simulink model "ROPOD_Control_SIM"  (R2017b)
settings: Solver=VariableStepAuto  StartTime=0.0  StopTime=inf  RelTol=1e-3
values from neighbouring files (symbols this model uses):
  AgentNumber = 1    [init_model.m]
  FFtheta_intia = 0    [init_model.m]
  FFxy_mass = 0*80    (= 0)    [init_model.m]
  flock_FFtheta_friction = 50    [init_model.m]
  flock_FFxy_friction = 100    [init_model.m]
  I_fhz_ddelta_cntr = 0    [init_model.m]
  I_fhz_dtheta_cntr = 0.3    [init_model.m]
  I_fhz_dtheta_flock_cntr = 0.1    [init_model.m]
  I_fhz_dvarphi_cntr = 0    [init_model.m]
  I_fhz_dxdy_cntr = 0.25    [init_model.m]
  I_fhz_dxdy_flock_cntr = 0.1    [init_model.m]
  K_gain_ddelta_cntr = 0.1    [init_model.m]
  K_gain_dtheta_cntr = 150    [init_model.m]
  K_gain_dtheta_flock_cntr = 100    [init_model.m]
  K_gain_dvarphi_cntr = 0.05    [init_model.m]
  K_gain_dxdy_cntr = 200    [init_model.m]
  K_gain_dxdy_flock_cntr = 200    [init_model.m]
  LL_wp_fhz_ddelta_cntr = 2    [init_model.m]
  LL_wp_fhz_dtheta_cntr = 20    [init_model.m]
  LL_wp_fhz_dtheta_flock_cntr = 20    [init_model.m]
  LL_wp_fhz_dvarphi_cntr = 10    [init_model.m]
  LL_wp_fhz_dxdy_cntr = 20    [init_model.m]
  LL_wp_fhz_dxdy_flock_cntr = 20    [init_model.m]
  LL_wz_fhz_ddelta_cntr = 2    [init_model.m]
  LL_wz_fhz_dtheta_cntr = 20    [init_model.m]
  LL_wz_fhz_dtheta_flock_cntr = 20    [init_model.m]
  LL_wz_fhz_dvarphi_cntr = 2    [init_model.m]
  LL_wz_fhz_dxdy_cntr = 20    [init_model.m]
  LL_wz_fhz_dxdy_flock_cntr = 20    [init_model.m]
  LPF_fhz_ddelta_cntr = 50    [init_model.m]
  LPF_fhz_ddelta_meas = 50    [init_model.m]
  LPF_fhz_dtheta_cntr = 100    [init_model.m]
  LPF_fhz_dtheta_flock_cntr = 40    [init_model.m]
  LPF_fhz_dvarphi_cntr = 50    [init_model.m]
  LPF_fhz_dvarphi_meas = 50    [init_model.m]
  LPF_fhz_dxdy_cntr = 100    [init_model.m]
  LPF_fhz_dxdy_flock_cntr = 40    [init_model.m]
  max_flock_acc_theta = 0.5    [init_model.m]
  max_flock_acc_xy = 0.5    [init_model.m]
  max_flock_vel_theta = 1.0    (= 1)    [init_model.m]
  max_flock_vel_xy = 1.0    (= 1)    [init_model.m]
  max_hw_tau = 7.0    (= 7)    [init_model.m]
  max_ropod_acc_theta = 1.6    [init_model.m]
  max_ropod_acc_xy = 2.0    (= 2)    [init_model.m]
  max_ropod_sw_force = 500    [init_model.m]
  max_ropod_sw_tau = 250    [init_model.m]
  max_ropod_vel_theta = 1.6    [init_model.m]
  max_ropod_vel_xy = 2.0    (= 2)    [init_model.m]
  max_sw_current = 10    [init_model.m]
  Nagents = 2    [init_model.m]
  Nwheels = 4    [Jqwl_numeric_function.m]    (also in S_matrix.m; extract_kinmodel_parameters.m; init_model.m; tau_optimal_dist_vec_fun.m)
  pivot_offs_sws = [0.0243    0.4689    0.3384    5.9050]    [init_model.m]
  ropod_kinmodel_pv = struct2array(ropod_kinmodel_param)    [set_ropod_KinModparams.m]
  ropod_position_inflock = [-1 0 3.1416]    [init_model.m]
  SW_COM1_ENABLE1 = hex2dec('0001')    [init_model.m]
  SW_COM1_ENABLE2 = hex2dec('0002')    [init_model.m]
  SW_COM1_MODE_TORQUE = bitshift(hex2dec('0000'),2)    [init_model.m]
  SW_COM1_MODE_VELOCITY = bitshift(hex2dec('0002'),2)    [init_model.m]
  SW_COM1_USE_TS = hex2dec('8000')    [init_model.m]
  sw_tau_2_current = 1/motor_physical_parameters.torqueconstant.value    [init_model.m]
  Tinit = 2    [init_model.m]
  Ts = 0.001    [init_model.m]
  Ts_MPC = 0.01    [init_model.m]
  Tsflck = 0.01    [init_model.m]
undefined symbols (not defined in the file or in its folder): acc_limit, accmax, b_cx, b_cy, b_rx, bus_size, comp_enable, Desired, DiscIntNeverNeededParam, Fcgain, gdis, k_cx, k_cy, live_tuning, m_robot, Nominal, Nominal_x, Nominal_y, offsets, portwidth, sizes, types, vel_limit, vmax1, vmax2
libraries: simulink x90, cstblocks x66, dspsigops x12, dspnetwork x4
(part 5 of 8)

== system ROPOD_Control_SIM/FlockController/Flock Velocity controller/G_I_LL_LPF Controller_flock_Y/Shapeit Lead-Lag (Tustin) ==
  In : Inport
  fz : Inport  Port=2
  fp : Inport  Port=3
  Add : Sum  Inputs=+-
  Constant1 : Constant
  Constant2 : Constant  Value=0
  Constant4 : Constant
  Divide : Product  Inputs=*/
  Divide1 : Product  Inputs=/*
  Gain1 : Gain  Gain=2*pi
  Gain2 : Gain  Gain=2*pi
  PID Controller3 : simulink/Continuous/PID Controller  Controller=PID  TimeDomain=Discrete-time  SampleTime=Tsflck  IntegratorMethod=Trapezoidal  FilterMethod=Trapezoidal  Form=Parallel  UseFilter=on  ControllerParametersSource=external  P=0.4  I=0.4*2*pi*3  D=0  N=100  InitialConditionSource=internal  InitialConditionForIntegrator=0  InitialConditionForFilter=0  ExternalReset=none  LimitOutput=off  UpperSaturationLimit=max_hw_tau  LowerSaturationLimit=-max_hw_tau  LinearizeAsGain=on  AntiWindupMode=clamping  Kb=1  TrackingMode=off  Kt=1  PParamMin=[]  PParamMax=[]  IParamMin=[]  IParamMax=[]  DParamMin=[]  DParamMax=[]  NParamMin=[]  NParamMax=[]  KbParamMin=[]  KbParamMax=[]  KtParamMin=[]  KtParamMax=[]  POutMin=[]  POutMax=[]  IOutMin=[]  IOutMax=[]  DOutMin=[]  DOutMax=[]  NOutMin=[]  NOutMax=[]  KbOutMin=[]  KbOutMax=[]  KtOutMin=[]  KtOutMax=[]  IntegratorOutMin=[]  IntegratorOutMax=[]  FilterOutMin=[]  FilterOutMax=[]  SumOutMin=[]  SumOutMax=[]  SumI1OutMin=[]  SumI1OutMax=[]  SumI2OutMin=[]  SumI2OutMax=[]  SumI3OutMin=[]  SumI3OutMax=[]  SumDOutMin=[]  SumDOutMax=[]  SaturationOutMin=[]  SaturationOutMax=[]  IntegratorContinuousStateAttributes=''  IntegratorStateMustResolveToSignalObject=off  IntegratorRTWStateStorageClass=Auto  FilterContinuousStateAttributes=''  FilterStateMustResolveToSignalObject=off  FilterRTWStateStorageClass=Auto  DifferentiatorICPrevScaledInput=0  DifferentiatorOutMin=[]  DifferentiatorOutMax=[]  InitialConditionSetting=State (most efficient)  FilterDiffOutCoefMin=[]  FilterDiffOutCoefMax=[]  SumDenOutMin=[]  SumDenOutMax=[]  SumNumOutMin=[]  SumNumOutMax=[]  ReciprocalOutMin=[]  ReciprocalOutMax=[]  DivideOutMin=[]  DivideOutMax=[]  TunerSelectOption=Transfer Function Based (PID Tuner App)
  Out : Outport
  wires:
  Constant4/1 -> PID Controller3/2
  In/1 -> PID Controller3/1
  PID Controller3/1 -> Out/1
  fz/1 -> Gain2/1
  fp/1 -> Gain1/1
  Gain1/1 -> PID Controller3/5, Divide/2
  Constant2/1 -> PID Controller3/3
  Gain2/1 -> Divide1/1, Divide/1
  Divide/1 -> Add/2
  Constant1/1 -> Add/1
  Add/1 -> Divide1/2
  Divide1/1 -> PID Controller3/4

== system ROPOD_Control_SIM/RopodTorqueDistribution/ROPOD 4SW/ROPOD_4Wheel_sens_own_vel_filter/Glitch removal + LP filter ==
  encoder : Inport
  LPF_fhz : Inport  Port=2
  Constant3 : Constant  Value=Ts
  Discrete Derivative : simulink/Discrete/Discrete Derivative  gainval=1  ICPrevScaledInput=0.0  OutMin=[]  OutMax=[]  OutDataType=fixdt(1, 16)  OutScaling=2^-10  DoSatur=off
  Discrete Varying Lowpass12 : cstblocks/Linear Parameter Varying/Discrete Varying Lowpass  N=2  w0=0  Ts=Ts
      settings: SourceProductName=Control System Toolbox  SourceProductBaseCode=CT
  Remove_glitches1 : MATLAB Function  TreatAsAtomicUnit=on
  Unit Delay : UnitDelay  SampleTime=-1
  Unwrap11 : dspsigops/Unwrap  tol=0.1  running=on
  sign convention4 : Gain  Gain=2*pi
  out : Outport
  wires:
  Unit Delay/1 -> Remove_glitches1/1(vel)
  sign convention4/1 -> Discrete Varying Lowpass12/2
  Unwrap11/1 -> Remove_glitches1/3(encoder)
  LPF_fhz/1 -> sign convention4/1
  Remove_glitches1/1(encoder_out) -> Discrete Derivative/1
  Constant3/1 -> Remove_glitches1/2(Ts)
  Discrete Varying Lowpass12/1 -> out/1
  encoder/1 -> Unwrap11/1
  Discrete Derivative/1 -> Unit Delay/1, Discrete Varying Lowpass12/1

== system ROPOD_Control_SIM/RopodTorqueDistribution/ROPOD 4SW/ROPOD_4Wheel_sens_own_vel_filter/Glitch removal + LP filter1 ==
  encoder : Inport
  LPF_fhz : Inport  Port=2
  Constant3 : Constant  Value=Ts
  Discrete Derivative : simulink/Discrete/Discrete Derivative  gainval=1  ICPrevScaledInput=0.0  OutMin=[]  OutMax=[]  OutDataType=fixdt(1, 16)  OutScaling=2^-10  DoSatur=off
  Discrete Varying Lowpass12 : cstblocks/Linear Parameter Varying/Discrete Varying Lowpass  N=2  w0=0  Ts=Ts
      settings: SourceProductName=Control System Toolbox  SourceProductBaseCode=CT
  Remove_glitches1 : MATLAB Function  TreatAsAtomicUnit=on
  Unit Delay : UnitDelay  SampleTime=-1
  Unwrap11 : dspsigops/Unwrap  tol=0.1  running=on
  sign convention4 : Gain  Gain=2*pi
  out : Outport
  wires:
  Discrete Derivative/1 -> Discrete Varying Lowpass12/1, Unit Delay/1
  encoder/1 -> Unwrap11/1
  Discrete Varying Lowpass12/1 -> out/1
  Constant3/1 -> Remove_glitches1/2(Ts)
  Remove_glitches1/1(encoder_out) -> Discrete Derivative/1
  LPF_fhz/1 -> sign convention4/1
  Unwrap11/1 -> Remove_glitches1/3(encoder)
  sign convention4/1 -> Discrete Varying Lowpass12/2
  Unit Delay/1 -> Remove_glitches1/1(vel)

== system ROPOD_Control_SIM/RopodTorqueDistribution/ROPOD 4SW/ROPOD_4Wheel_sens_own_vel_filter/Glitch removal + LP filter10 ==
  encoder : Inport
  LPF_fhz : Inport  Port=2
  Constant3 : Constant  Value=Ts
  Discrete Derivative : simulink/Discrete/Discrete Derivative  gainval=1  ICPrevScaledInput=0.0  OutMin=[]  OutMax=[]  OutDataType=fixdt(1, 16)  OutScaling=2^-10  DoSatur=off
  Discrete Varying Lowpass12 : cstblocks/Linear Parameter Varying/Discrete Varying Lowpass  N=2  w0=0  Ts=Ts
      settings: SourceProductName=Control System Toolbox  SourceProductBaseCode=CT
  Remove_glitches1 : MATLAB Function  TreatAsAtomicUnit=on
  Unit Delay : UnitDelay  SampleTime=-1
  Unwrap11 : dspsigops/Unwrap  tol=0.1  running=on
  sign convention4 : Gain  Gain=2*pi
  enc_out : Outport
  out : Outport  Port=2
  wires:
  Unit Delay/1 -> Remove_glitches1/1(vel)
  sign convention4/1 -> Discrete Varying Lowpass12/2
  Unwrap11/1 -> Remove_glitches1/3(encoder)
  LPF_fhz/1 -> sign convention4/1
  Remove_glitches1/1(encoder_out) -> enc_out/1, Discrete Derivative/1
  Constant3/1 -> Remove_glitches1/2(Ts)
  Discrete Varying Lowpass12/1 -> out/1
  encoder/1 -> Unwrap11/1
  Discrete Derivative/1 -> Unit Delay/1, Discrete Varying Lowpass12/1

== system ROPOD_Control_SIM/RopodTorqueDistribution/ROPOD 4SW/ROPOD_4Wheel_sens_own_vel_filter/Glitch removal + LP filter11 ==
  encoder : Inport
  LPF_fhz : Inport  Port=2
  Constant3 : Constant  Value=Ts
  Discrete Derivative : simulink/Discrete/Discrete Derivative  gainval=1  ICPrevScaledInput=0.0  OutMin=[]  OutMax=[]  OutDataType=fixdt(1, 16)  OutScaling=2^-10  DoSatur=off
  Discrete Varying Lowpass12 : cstblocks/Linear Parameter Varying/Discrete Varying Lowpass  N=2  w0=0  Ts=Ts
      settings: SourceProductName=Control System Toolbox  SourceProductBaseCode=CT
  Remove_glitches1 : MATLAB Function  TreatAsAtomicUnit=on
  Unit Delay : UnitDelay  SampleTime=-1
  Unwrap11 : dspsigops/Unwrap  tol=0.1  running=on
  sign convention4 : Gain  Gain=2*pi
  encoder_out : Outport
  vel_out : Outport  Port=2
  wires:
  Unit Delay/1 -> Remove_glitches1/1(vel)
  sign convention4/1 -> Discrete Varying Lowpass12/2
  Unwrap11/1 -> Remove_glitches1/3(encoder)
  LPF_fhz/1 -> sign convention4/1
  Remove_glitches1/1(encoder_out) -> encoder_out/1, Discrete Derivative/1
  Constant3/1 -> Remove_glitches1/2(Ts)
  Discrete Varying Lowpass12/1 -> vel_out/1
  encoder/1 -> Unwrap11/1
  Discrete Derivative/1 -> Unit Delay/1, Discrete Varying Lowpass12/1

== system ROPOD_Control_SIM/RopodTorqueDistribution/ROPOD 4SW/ROPOD_4Wheel_sens_own_vel_filter/Glitch removal + LP filter2 ==
  encoder : Inport
  LPF_fhz : Inport  Port=2
  Constant3 : Constant  Value=Ts
  Discrete Derivative : simulink/Discrete/Discrete Derivative  gainval=1  ICPrevScaledInput=0.0  OutMin=[]  OutMax=[]  OutDataType=fixdt(1, 16)  OutScaling=2^-10  DoSatur=off
  Discrete Varying Lowpass12 : cstblocks/Linear Parameter Varying/Discrete Varying Lowpass  N=2  w0=0  Ts=Ts
      settings: SourceProductName=Control System Toolbox  SourceProductBaseCode=CT
  Remove_glitches1 : MATLAB Function  TreatAsAtomicUnit=on
  Unit Delay : UnitDelay  SampleTime=-1
  Unwrap11 : dspsigops/Unwrap  tol=0.1  running=on
  sign convention4 : Gain  Gain=2*pi
  encoder_out : Outport
  vel_out : Outport  Port=2
  wires:
  Unit Delay/1 -> Remove_glitches1/1(vel)
  sign convention4/1 -> Discrete Varying Lowpass12/2
  Unwrap11/1 -> Remove_glitches1/3(encoder)
  LPF_fhz/1 -> sign convention4/1
  Remove_glitches1/1(encoder_out) -> encoder_out/1, Discrete Derivative/1
  Constant3/1 -> Remove_glitches1/2(Ts)
  Discrete Varying Lowpass12/1 -> vel_out/1
  encoder/1 -> Unwrap11/1
  Discrete Derivative/1 -> Unit Delay/1, Discrete Varying Lowpass12/1

== system ROPOD_Control_SIM/RopodTorqueDistribution/ROPOD 4SW/ROPOD_4Wheel_sens_own_vel_filter/Glitch removal + LP filter3 ==
  encoder : Inport
  LPF_fhz : Inport  Port=2
  Constant3 : Constant  Value=Ts
  Discrete Derivative : simulink/Discrete/Discrete Derivative  gainval=1  ICPrevScaledInput=0.0  OutMin=[]  OutMax=[]  OutDataType=fixdt(1, 16)  OutScaling=2^-10  DoSatur=off
  Discrete Varying Lowpass12 : cstblocks/Linear Parameter Varying/Discrete Varying Lowpass  N=2  w0=0  Ts=Ts
      settings: SourceProductName=Control System Toolbox  SourceProductBaseCode=CT
  Remove_glitches1 : MATLAB Function  TreatAsAtomicUnit=on
  Unit Delay : UnitDelay  SampleTime=-1
  Unwrap11 : dspsigops/Unwrap  tol=0.1  running=on
  sign convention4 : Gain  Gain=2*pi
  out : Outport
  wires:
  Unit Delay/1 -> Remove_glitches1/1(vel)
  sign convention4/1 -> Discrete Varying Lowpass12/2
  Unwrap11/1 -> Remove_glitches1/3(encoder)
  LPF_fhz/1 -> sign convention4/1
  Remove_glitches1/1(encoder_out) -> Discrete Derivative/1
  Constant3/1 -> Remove_glitches1/2(Ts)
  Discrete Varying Lowpass12/1 -> out/1
  encoder/1 -> Unwrap11/1
  Discrete Derivative/1 -> Unit Delay/1, Discrete Varying Lowpass12/1

== system ROPOD_Control_SIM/RopodTorqueDistribution/ROPOD 4SW/ROPOD_4Wheel_sens_own_vel_filter/Glitch removal + LP filter4 ==
  encoder : Inport
  LPF_fhz : Inport  Port=2
  Constant3 : Constant  Value=Ts
  Discrete Derivative : simulink/Discrete/Discrete Derivative  gainval=1  ICPrevScaledInput=0.0  OutMin=[]  OutMax=[]  OutDataType=fixdt(1, 16)  OutScaling=2^-10  DoSatur=off
  Discrete Varying Lowpass12 : cstblocks/Linear Parameter Varying/Discrete Varying Lowpass  N=2  w0=0  Ts=Ts
      settings: SourceProductName=Control System Toolbox  SourceProductBaseCode=CT
  Remove_glitches1 : MATLAB Function  TreatAsAtomicUnit=on
  Unit Delay : UnitDelay  SampleTime=-1
  Unwrap11 : dspsigops/Unwrap  tol=0.1  running=on
  sign convention4 : Gain  Gain=2*pi
  out : Outport
  wires:
  Discrete Derivative/1 -> Discrete Varying Lowpass12/1, Unit Delay/1
  encoder/1 -> Unwrap11/1
  Discrete Varying Lowpass12/1 -> out/1
  Constant3/1 -> Remove_glitches1/2(Ts)
  Remove_glitches1/1(encoder_out) -> Discrete Derivative/1
  LPF_fhz/1 -> sign convention4/1
  Unwrap11/1 -> Remove_glitches1/3(encoder)
  sign convention4/1 -> Discrete Varying Lowpass12/2
  Unit Delay/1 -> Remove_glitches1/1(vel)

== system ROPOD_Control_SIM/RopodTorqueDistribution/ROPOD 4SW/ROPOD_4Wheel_sens_own_vel_filter/Glitch removal + LP filter5 ==
  encoder : Inport
  LPF_fhz : Inport  Port=2
  Constant3 : Constant  Value=Ts
  Discrete Derivative : simulink/Discrete/Discrete Derivative  gainval=1  ICPrevScaledInput=0.0  OutMin=[]  OutMax=[]  OutDataType=fixdt(1, 16)  OutScaling=2^-10  DoSatur=off
  Discrete Varying Lowpass12 : cstblocks/Linear Parameter Varying/Discrete Varying Lowpass  N=2  w0=0  Ts=Ts
      settings: SourceProductName=Control System Toolbox  SourceProductBaseCode=CT
  Remove_glitches1 : MATLAB Function  TreatAsAtomicUnit=on
  Unit Delay : UnitDelay  SampleTime=-1
  Unwrap11 : dspsigops/Unwrap  tol=0.1  running=on
  sign convention4 : Gain  Gain=2*pi
  encoder_out : Outport
  vel_out : Outport  Port=2
  wires:
  Unit Delay/1 -> Remove_glitches1/1(vel)
  sign convention4/1 -> Discrete Varying Lowpass12/2
  Unwrap11/1 -> Remove_glitches1/3(encoder)
  LPF_fhz/1 -> sign convention4/1
  Remove_glitches1/1(encoder_out) -> encoder_out/1, Discrete Derivative/1
  Constant3/1 -> Remove_glitches1/2(Ts)
  Discrete Varying Lowpass12/1 -> vel_out/1
  encoder/1 -> Unwrap11/1
  Discrete Derivative/1 -> Unit Delay/1, Discrete Varying Lowpass12/1

== system ROPOD_Control_SIM/RopodTorqueDistribution/ROPOD 4SW/ROPOD_4Wheel_sens_own_vel_filter/Glitch removal + LP filter6 ==
  encoder : Inport
  LPF_fhz : Inport  Port=2
  Constant3 : Constant  Value=Ts
  Discrete Derivative : simulink/Discrete/Discrete Derivative  gainval=1  ICPrevScaledInput=0.0  OutMin=[]  OutMax=[]  OutDataType=fixdt(1, 16)  OutScaling=2^-10  DoSatur=off
  Discrete Varying Lowpass12 : cstblocks/Linear Parameter Varying/Discrete Varying Lowpass  N=2  w0=0  Ts=Ts
      settings: SourceProductName=Control System Toolbox  SourceProductBaseCode=CT
  Remove_glitches1 : MATLAB Function  TreatAsAtomicUnit=on
  Unit Delay : UnitDelay  SampleTime=-1
  Unwrap11 : dspsigops/Unwrap  tol=0.1  running=on
  sign convention4 : Gain  Gain=2*pi
  out : Outport
  wires:
  Unit Delay/1 -> Remove_glitches1/1(vel)
  sign convention4/1 -> Discrete Varying Lowpass12/2
  Unwrap11/1 -> Remove_glitches1/3(encoder)
  LPF_fhz/1 -> sign convention4/1
  Remove_glitches1/1(encoder_out) -> Discrete Derivative/1
  Constant3/1 -> Remove_glitches1/2(Ts)
  Discrete Varying Lowpass12/1 -> out/1
  encoder/1 -> Unwrap11/1
  Discrete Derivative/1 -> Unit Delay/1, Discrete Varying Lowpass12/1

== system ROPOD_Control_SIM/RopodTorqueDistribution/ROPOD 4SW/ROPOD_4Wheel_sens_own_vel_filter/Glitch removal + LP filter7 ==
  encoder : Inport
  LPF_fhz : Inport  Port=2
  Constant3 : Constant  Value=Ts
  Discrete Derivative : simulink/Discrete/Discrete Derivative  gainval=1  ICPrevScaledInput=0.0  OutMin=[]  OutMax=[]  OutDataType=fixdt(1, 16)  OutScaling=2^-10  DoSatur=off
  Discrete Varying Lowpass12 : cstblocks/Linear Parameter Varying/Discrete Varying Lowpass  N=2  w0=0  Ts=Ts
      settings: SourceProductName=Control System Toolbox  SourceProductBaseCode=CT
  Remove_glitches1 : MATLAB Function  TreatAsAtomicUnit=on
  Unit Delay : UnitDelay  SampleTime=-1
  Unwrap11 : dspsigops/Unwrap  tol=0.1  running=on
  sign convention4 : Gain  Gain=2*pi
  out : Outport
  wires:
  Discrete Derivative/1 -> Discrete Varying Lowpass12/1, Unit Delay/1
  encoder/1 -> Unwrap11/1
  Discrete Varying Lowpass12/1 -> out/1
  Constant3/1 -> Remove_glitches1/2(Ts)
  Remove_glitches1/1(encoder_out) -> Discrete Derivative/1
  LPF_fhz/1 -> sign convention4/1
  Unwrap11/1 -> Remove_glitches1/3(encoder)
  sign convention4/1 -> Discrete Varying Lowpass12/2
  Unit Delay/1 -> Remove_glitches1/1(vel)

== system ROPOD_Control_SIM/RopodTorqueDistribution/ROPOD 4SW/ROPOD_4Wheel_sens_own_vel_filter/Glitch removal + LP filter8 ==
  encoder : Inport
  LPF_fhz : Inport  Port=2
  Constant3 : Constant  Value=Ts
  Discrete Derivative : simulink/Discrete/Discrete Derivative  gainval=1  ICPrevScaledInput=0.0  OutMin=[]  OutMax=[]  OutDataType=fixdt(1, 16)  OutScaling=2^-10  DoSatur=off
  Discrete Varying Lowpass12 : cstblocks/Linear Parameter Varying/Discrete Varying Lowpass  N=2  w0=0  Ts=Ts
      settings: SourceProductName=Control System Toolbox  SourceProductBaseCode=CT
  Remove_glitches1 : MATLAB Function  TreatAsAtomicUnit=on
  Unit Delay : UnitDelay  SampleTime=-1
  Unwrap11 : dspsigops/Unwrap  tol=0.1  running=on
  sign convention4 : Gain  Gain=2*pi
  encoder_out : Outport
  vel_out : Outport  Port=2
  wires:
  Unit Delay/1 -> Remove_glitches1/1(vel)
  sign convention4/1 -> Discrete Varying Lowpass12/2
  Unwrap11/1 -> Remove_glitches1/3(encoder)
  LPF_fhz/1 -> sign convention4/1
  Remove_glitches1/1(encoder_out) -> encoder_out/1, Discrete Derivative/1
  Constant3/1 -> Remove_glitches1/2(Ts)
  Discrete Varying Lowpass12/1 -> vel_out/1
  encoder/1 -> Unwrap11/1
  Discrete Derivative/1 -> Unit Delay/1, Discrete Varying Lowpass12/1

== system ROPOD_Control_SIM/RopodTorqueDistribution/ROPOD 4SW/ROPOD_4Wheel_sens_own_vel_filter/Glitch removal + LP filter9 ==
  encoder : Inport
  LPF_fhz : Inport  Port=2
  Constant3 : Constant  Value=Ts
  Discrete Derivative : simulink/Discrete/Discrete Derivative  gainval=1  ICPrevScaledInput=0.0  OutMin=[]  OutMax=[]  OutDataType=fixdt(1, 16)  OutScaling=2^-10  DoSatur=off
  Discrete Varying Lowpass12 : cstblocks/Linear Parameter Varying/Discrete Varying Lowpass  N=2  w0=0  Ts=Ts
      settings: SourceProductName=Control System Toolbox  SourceProductBaseCode=CT
  Remove_glitches1 : MATLAB Function  TreatAsAtomicUnit=on
  Unit Delay : UnitDelay  SampleTime=-1
  Unwrap11 : dspsigops/Unwrap  tol=0.1  running=on
  sign convention4 : Gain  Gain=2*pi
  enc_out : Outport
  out : Outport  Port=2
  wires:
  Unit Delay/1 -> Remove_glitches1/1(vel)
  sign convention4/1 -> Discrete Varying Lowpass12/2
  Unwrap11/1 -> Remove_glitches1/3(encoder)
  LPF_fhz/1 -> sign convention4/1
  Remove_glitches1/1(encoder_out) -> enc_out/1, Discrete Derivative/1
  Constant3/1 -> Remove_glitches1/2(Ts)
  Discrete Varying Lowpass12/1 -> out/1
  encoder/1 -> Unwrap11/1
  Discrete Derivative/1 -> Unit Delay/1, Discrete Varying Lowpass12/1

== system ROPOD_Control_SIM/RopodTorqueDistribution/pivot damping cntr/Pivot controller/G_I_LL_LPF Controller1 ==
  param : Inport
  In : Inport  Port=2
  reset_integrator : Inport  Port=3
  Bus Selector : BusSelector  OutputSignals=P_gain,I_freq_hz,LL_zero_fhz,LL_pole_fhz,LPF_fhz
  Discrete Varying Lowpass3 : cstblocks/Linear Parameter Varying/Discrete Varying Lowpass  N=1  w0=0  Ts=Ts
      settings: SourceProductName=Control System Toolbox  SourceProductBaseCode=CT
  Gain2 : Gain  Gain=2*pi
  Product5 : Product
  Shapeit Integrator (Tustin) : Subsystem
  Shapeit Lead-Lag (Tustin) : Subsystem
  Out : Outport
  wires:
  Gain2/1 -> Discrete Varying Lowpass3/2
  Product5/1 -> Shapeit Integrator (Tustin)/1(In)
  Discrete Varying Lowpass3/1 -> Out/1
  Shapeit Integrator (Tustin)/1(Out) -> Shapeit Lead-Lag (Tustin)/1(In)
  Bus Selector/1 -> Product5/2  "<P_gain>"
  Bus Selector/2 -> Shapeit Integrator (Tustin)/2(I_fhz)  "<I_freq_hz>"
  param/1 -> Bus Selector/1
  Bus Selector/5 -> Gain2/1  "<LPF_fhz>"
  Bus Selector/4 -> Shapeit Lead-Lag (Tustin)/3(fp)  "<LL_pole_fhz>"
  reset_integrator/1 -> Shapeit Integrator (Tustin)/3(reset)
  Bus Selector/3 -> Shapeit Lead-Lag (Tustin)/2(fz)  "<LL_zero_fhz>"
  Shapeit Lead-Lag (Tustin)/1(Out) -> Discrete Varying Lowpass3/1
  In/1 -> Product5/1

== system ROPOD_Control_SIM/RopodTorqueDistribution/pivot damping cntr/Pivot controller/G_I_LL_LPF Controller2 ==
  param : Inport
  In : Inport  Port=2
  reset_integrator : Inport  Port=3
  Bus Selector : BusSelector  OutputSignals=P_gain,I_freq_hz,LL_zero_fhz,LL_pole_fhz,LPF_fhz
  Discrete Varying Lowpass3 : cstblocks/Linear Parameter Varying/Discrete Varying Lowpass  N=1  w0=0  Ts=Ts
      settings: SourceProductName=Control System Toolbox  SourceProductBaseCode=CT
  Gain2 : Gain  Gain=2*pi
  Product5 : Product
  Shapeit Integrator (Tustin) : Subsystem
  Shapeit Lead-Lag (Tustin) : Subsystem
  Out : Outport
  wires:
  Gain2/1 -> Discrete Varying Lowpass3/2
  Product5/1 -> Shapeit Integrator (Tustin)/1(In)
  Discrete Varying Lowpass3/1 -> Out/1
  Shapeit Integrator (Tustin)/1(Out) -> Shapeit Lead-Lag (Tustin)/1(In)
  Bus Selector/1 -> Product5/2  "<P_gain>"
  Bus Selector/2 -> Shapeit Integrator (Tustin)/2(I_fhz)  "<I_freq_hz>"
  param/1 -> Bus Selector/1
  Bus Selector/5 -> Gain2/1  "<LPF_fhz>"
  Bus Selector/4 -> Shapeit Lead-Lag (Tustin)/3(fp)  "<LL_pole_fhz>"
  reset_integrator/1 -> Shapeit Integrator (Tustin)/3(reset)
  Bus Selector/3 -> Shapeit Lead-Lag (Tustin)/2(fz)  "<LL_zero_fhz>"
  Shapeit Lead-Lag (Tustin)/1(Out) -> Discrete Varying Lowpass3/1
  In/1 -> Product5/1

== system ROPOD_Control_SIM/RopodTorqueDistribution/pivot damping cntr/Pivot controller/G_I_LL_LPF Controller3 ==
  param : Inport
  In : Inport  Port=2
  reset_integrator : Inport  Port=3
  Bus Selector : BusSelector  OutputSignals=P_gain,I_freq_hz,LL_zero_fhz,LL_pole_fhz,LPF_fhz
  Discrete Varying Lowpass3 : cstblocks/Linear Parameter Varying/Discrete Varying Lowpass  N=1  w0=0  Ts=Ts
      settings: SourceProductName=Control System Toolbox  SourceProductBaseCode=CT
  Gain2 : Gain  Gain=2*pi
  Product5 : Product
  Shapeit Integrator (Tustin) : Subsystem
  Shapeit Lead-Lag (Tustin) : Subsystem
  Out : Outport
  wires:
  In/1 -> Product5/1
  Shapeit Lead-Lag (Tustin)/1(Out) -> Discrete Varying Lowpass3/1
  Bus Selector/3 -> Shapeit Lead-Lag (Tustin)/2(fz)  "<LL_zero_fhz>"
  reset_integrator/1 -> Shapeit Integrator (Tustin)/3(reset)
  Bus Selector/4 -> Shapeit Lead-Lag (Tustin)/3(fp)  "<LL_pole_fhz>"
  Bus Selector/5 -> Gain2/1  "<LPF_fhz>"
  param/1 -> Bus Selector/1
  Bus Selector/2 -> Shapeit Integrator (Tustin)/2(I_fhz)  "<I_freq_hz>"
  Bus Selector/1 -> Product5/2  "<P_gain>"
  Shapeit Integrator (Tustin)/1(Out) -> Shapeit Lead-Lag (Tustin)/1(In)
  Discrete Varying Lowpass3/1 -> Out/1
  Product5/1 -> Shapeit Integrator (Tustin)/1(In)
  Gain2/1 -> Discrete Varying Lowpass3/2

== system ROPOD_Control_SIM/RopodTorqueDistribution/pivot damping cntr/Pivot controller/G_I_LL_LPF Controller4 ==
  param : Inport
  In : Inport  Port=2
  reset_integrator : Inport  Port=3
  Bus Selector : BusSelector  OutputSignals=P_gain,I_freq_hz,LL_zero_fhz,LL_pole_fhz,LPF_fhz
  Discrete Varying Lowpass3 : cstblocks/Linear Parameter Varying/Discrete Varying Lowpass  N=1  w0=0  Ts=Ts
      settings: SourceProductName=Control System Toolbox  SourceProductBaseCode=CT
  Gain2 : Gain  Gain=2*pi
  Product5 : Product
  Shapeit Integrator (Tustin) : Subsystem
  Shapeit Lead-Lag (Tustin) : Subsystem
  Out : Outport
  wires:
  Gain2/1 -> Discrete Varying Lowpass3/2
  Product5/1 -> Shapeit Integrator (Tustin)/1(In)
  Discrete Varying Lowpass3/1 -> Out/1
  Shapeit Integrator (Tustin)/1(Out) -> Shapeit Lead-Lag (Tustin)/1(In)
  Bus Selector/1 -> Product5/2  "<P_gain>"
  Bus Selector/2 -> Shapeit Integrator (Tustin)/2(I_fhz)  "<I_freq_hz>"
  param/1 -> Bus Selector/1
  Bus Selector/5 -> Gain2/1  "<LPF_fhz>"
  Bus Selector/4 -> Shapeit Lead-Lag (Tustin)/3(fp)  "<LL_pole_fhz>"
  reset_integrator/1 -> Shapeit Integrator (Tustin)/3(reset)
  Bus Selector/3 -> Shapeit Lead-Lag (Tustin)/2(fz)  "<LL_zero_fhz>"
  Shapeit Lead-Lag (Tustin)/1(Out) -> Discrete Varying Lowpass3/1
  In/1 -> Product5/1

== system ROPOD_Control_SIM/RopodTorqueDistribution/wheel vel cntr/Wheels Velocity controller/G_I_LL_LPF Controller1 ==
  param : Inport
  In : Inport  Port=2
  reset_integrator : Inport  Port=3
  Bus Selector : BusSelector  OutputSignals=P_gain,I_freq_hz,LL_zero_fhz,LL_pole_fhz,LPF_fhz
  Discrete Varying Lowpass3 : cstblocks/Linear Parameter Varying/Discrete Varying Lowpass  N=1  w0=0  Ts=Ts
      settings: SourceProductName=Control System Toolbox  SourceProductBaseCode=CT
  Gain2 : Gain  Gain=2*pi
  Product5 : Product
  Shapeit Integrator (Tustin) : Subsystem
  Shapeit Lead-Lag (Tustin) : Subsystem
  Out : Outport
  wires:
  Gain2/1 -> Discrete Varying Lowpass3/2
  Product5/1 -> Shapeit Integrator (Tustin)/1(In)
  Discrete Varying Lowpass3/1 -> Out/1
  Shapeit Integrator (Tustin)/1(Out) -> Shapeit Lead-Lag (Tustin)/1(In)
  Bus Selector/1 -> Product5/2  "<P_gain>"
  Bus Selector/2 -> Shapeit Integrator (Tustin)/2(I_fhz)  "<I_freq_hz>"
  param/1 -> Bus Selector/1
  Bus Selector/5 -> Gain2/1  "<LPF_fhz>"
  Bus Selector/4 -> Shapeit Lead-Lag (Tustin)/3(fp)  "<LL_pole_fhz>"
  reset_integrator/1 -> Shapeit Integrator (Tustin)/3(reset)
  Bus Selector/3 -> Shapeit Lead-Lag (Tustin)/2(fz)  "<LL_zero_fhz>"
  Shapeit Lead-Lag (Tustin)/1(Out) -> Discrete Varying Lowpass3/1
  In/1 -> Product5/1

== system ROPOD_Control_SIM/RopodTorqueDistribution/wheel vel cntr/Wheels Velocity controller/G_I_LL_LPF Controller2 ==
  param : Inport
  In : Inport  Port=2
  reset_integrator : Inport  Port=3
  Bus Selector : BusSelector  OutputSignals=P_gain,I_freq_hz,LL_zero_fhz,LL_pole_fhz,LPF_fhz
  Discrete Varying Lowpass3 : cstblocks/Linear Parameter Varying/Discrete Varying Lowpass  N=1  w0=0  Ts=Ts
      settings: SourceProductName=Control System Toolbox  SourceProductBaseCode=CT
  Gain2 : Gain  Gain=2*pi
  Product5 : Product
  Shapeit Integrator (Tustin) : Subsystem
  Shapeit Lead-Lag (Tustin) : Subsystem
  Out : Outport
  wires:
  Gain2/1 -> Discrete Varying Lowpass3/2
  Product5/1 -> Shapeit Integrator (Tustin)/1(In)
  Discrete Varying Lowpass3/1 -> Out/1
  Shapeit Integrator (Tustin)/1(Out) -> Shapeit Lead-Lag (Tustin)/1(In)
  Bus Selector/1 -> Product5/2  "<P_gain>"
  Bus Selector/2 -> Shapeit Integrator (Tustin)/2(I_fhz)  "<I_freq_hz>"
  param/1 -> Bus Selector/1
  Bus Selector/5 -> Gain2/1  "<LPF_fhz>"
  Bus Selector/4 -> Shapeit Lead-Lag (Tustin)/3(fp)  "<LL_pole_fhz>"
  reset_integrator/1 -> Shapeit Integrator (Tustin)/3(reset)
  Bus Selector/3 -> Shapeit Lead-Lag (Tustin)/2(fz)  "<LL_zero_fhz>"
  Shapeit Lead-Lag (Tustin)/1(Out) -> Discrete Varying Lowpass3/1
  In/1 -> Product5/1

== system ROPOD_Control_SIM/RopodTorqueDistribution/wheel vel cntr/Wheels Velocity controller/G_I_LL_LPF Controller3 ==
  param : Inport
  In : Inport  Port=2
  reset_integrator : Inport  Port=3
  Bus Selector : BusSelector  OutputSignals=P_gain,I_freq_hz,LL_zero_fhz,LL_pole_fhz,LPF_fhz
  Discrete Varying Lowpass3 : cstblocks/Linear Parameter Varying/Discrete Varying Lowpass  N=1  w0=0  Ts=Ts
      settings: SourceProductName=Control System Toolbox  SourceProductBaseCode=CT
  Gain2 : Gain  Gain=2*pi
  Product5 : Product
  Shapeit Integrator (Tustin) : Subsystem
  Shapeit Lead-Lag (Tustin) : Subsystem
  Out : Outport
  wires:
  In/1 -> Product5/1
  Shapeit Lead-Lag (Tustin)/1(Out) -> Discrete Varying Lowpass3/1
  Bus Selector/3 -> Shapeit Lead-Lag (Tustin)/2(fz)  "<LL_zero_fhz>"
  reset_integrator/1 -> Shapeit Integrator (Tustin)/3(reset)
  Bus Selector/4 -> Shapeit Lead-Lag (Tustin)/3(fp)  "<LL_pole_fhz>"
  Bus Selector/5 -> Gain2/1  "<LPF_fhz>"
  param/1 -> Bus Selector/1
  Bus Selector/2 -> Shapeit Integrator (Tustin)/2(I_fhz)  "<I_freq_hz>"
  Bus Selector/1 -> Product5/2  "<P_gain>"
  Shapeit Integrator (Tustin)/1(Out) -> Shapeit Lead-Lag (Tustin)/1(In)
  Discrete Varying Lowpass3/1 -> Out/1
  Product5/1 -> Shapeit Integrator (Tustin)/1(In)
  Gain2/1 -> Discrete Varying Lowpass3/2

== system ROPOD_Control_SIM/RopodTorqueDistribution/wheel vel cntr/Wheels Velocity controller/G_I_LL_LPF Controller4 ==
  param : Inport
  In : Inport  Port=2
  reset_integrator : Inport  Port=3
  Bus Selector : BusSelector  OutputSignals=P_gain,I_freq_hz,LL_zero_fhz,LL_pole_fhz,LPF_fhz
  Discrete Varying Lowpass3 : cstblocks/Linear Parameter Varying/Discrete Varying Lowpass  N=1  w0=0  Ts=Ts
      settings: SourceProductName=Control System Toolbox  SourceProductBaseCode=CT
  Gain2 : Gain  Gain=2*pi
  Product5 : Product
  Shapeit Integrator (Tustin) : Subsystem
  Shapeit Lead-Lag (Tustin) : Subsystem
  Out : Outport
  wires:
  Gain2/1 -> Discrete Varying Lowpass3/2
  Product5/1 -> Shapeit Integrator (Tustin)/1(In)
  Discrete Varying Lowpass3/1 -> Out/1
  Shapeit Integrator (Tustin)/1(Out) -> Shapeit Lead-Lag (Tustin)/1(In)
  Bus Selector/1 -> Product5/2  "<P_gain>"
  Bus Selector/2 -> Shapeit Integrator (Tustin)/2(I_fhz)  "<I_freq_hz>"
  param/1 -> Bus Selector/1
  Bus Selector/5 -> Gain2/1  "<LPF_fhz>"
  Bus Selector/4 -> Shapeit Lead-Lag (Tustin)/3(fp)  "<LL_pole_fhz>"
  reset_integrator/1 -> Shapeit Integrator (Tustin)/3(reset)
  Bus Selector/3 -> Shapeit Lead-Lag (Tustin)/2(fz)  "<LL_zero_fhz>"
  Shapeit Lead-Lag (Tustin)/1(Out) -> Discrete Varying Lowpass3/1
  In/1 -> Product5/1

== system ROPOD_Control_SIM/RopodTorqueDistribution/wheel vel cntr/Wheels Velocity controller/G_I_LL_LPF Controller5 ==
  param : Inport
  In : Inport  Port=2
  reset_integrator : Inport  Port=3
  Bus Selector : BusSelector  OutputSignals=P_gain,I_freq_hz,LL_zero_fhz,LL_pole_fhz,LPF_fhz
  Discrete Varying Lowpass3 : cstblocks/Linear Parameter Varying/Discrete Varying Lowpass  N=1  w0=0  Ts=Ts
      settings: SourceProductName=Control System Toolbox  SourceProductBaseCode=CT
  Gain2 : Gain  Gain=2*pi
  Product5 : Product
  Shapeit Integrator (Tustin) : Subsystem
  Shapeit Lead-Lag (Tustin) : Subsystem
  Out : Outport
  wires:
  In/1 -> Product5/1
  Shapeit Lead-Lag (Tustin)/1(Out) -> Discrete Varying Lowpass3/1
  Bus Selector/3 -> Shapeit Lead-Lag (Tustin)/2(fz)  "<LL_zero_fhz>"
  reset_integrator/1 -> Shapeit Integrator (Tustin)/3(reset)
  Bus Selector/4 -> Shapeit Lead-Lag (Tustin)/3(fp)  "<LL_pole_fhz>"
  Bus Selector/5 -> Gain2/1  "<LPF_fhz>"
  param/1 -> Bus Selector/1
  Bus Selector/2 -> Shapeit Integrator (Tustin)/2(I_fhz)  "<I_freq_hz>"
  Bus Selector/1 -> Product5/2  "<P_gain>"
  Shapeit Integrator (Tustin)/1(Out) -> Shapeit Lead-Lag (Tustin)/1(In)
  Discrete Varying Lowpass3/1 -> Out/1
  Product5/1 -> Shapeit Integrator (Tustin)/1(In)
  Gain2/1 -> Discrete Varying Lowpass3/2

== system ROPOD_Control_SIM/RopodTorqueDistribution/wheel vel cntr/Wheels Velocity controller/G_I_LL_LPF Controller6 ==
  param : Inport
  In : Inport  Port=2
  reset_integrator : Inport  Port=3
  Bus Selector : BusSelector  OutputSignals=P_gain,I_freq_hz,LL_zero_fhz,LL_pole_fhz,LPF_fhz
  Discrete Varying Lowpass3 : cstblocks/Linear Parameter Varying/Discrete Varying Lowpass  N=1  w0=0  Ts=Ts
      settings: SourceProductName=Control System Toolbox  SourceProductBaseCode=CT
  Gain2 : Gain  Gain=2*pi
  Product5 : Product
  Shapeit Integrator (Tustin) : Subsystem
  Shapeit Lead-Lag (Tustin) : Subsystem
  Out : Outport
  wires:
  Gain2/1 -> Discrete Varying Lowpass3/2
  Product5/1 -> Shapeit Integrator (Tustin)/1(In)
  Discrete Varying Lowpass3/1 -> Out/1
  Shapeit Integrator (Tustin)/1(Out) -> Shapeit Lead-Lag (Tustin)/1(In)
  Bus Selector/1 -> Product5/2  "<P_gain>"
  Bus Selector/2 -> Shapeit Integrator (Tustin)/2(I_fhz)  "<I_freq_hz>"
  param/1 -> Bus Selector/1
  Bus Selector/5 -> Gain2/1  "<LPF_fhz>"
  Bus Selector/4 -> Shapeit Lead-Lag (Tustin)/3(fp)  "<LL_pole_fhz>"
  reset_integrator/1 -> Shapeit Integrator (Tustin)/3(reset)
  Bus Selector/3 -> Shapeit Lead-Lag (Tustin)/2(fz)  "<LL_zero_fhz>"
  Shapeit Lead-Lag (Tustin)/1(Out) -> Discrete Varying Lowpass3/1
  In/1 -> Product5/1

== system ROPOD_Control_SIM/RopodTorqueDistribution/wheel vel cntr/Wheels Velocity controller/G_I_LL_LPF Controller7 ==
  param : Inport
  In : Inport  Port=2
  reset_integrator : Inport  Port=3
  Bus Selector : BusSelector  OutputSignals=P_gain,I_freq_hz,LL_zero_fhz,LL_pole_fhz,LPF_fhz
  Discrete Varying Lowpass3 : cstblocks/Linear Parameter Varying/Discrete Varying Lowpass  N=1  w0=0  Ts=Ts
      settings: SourceProductName=Control System Toolbox  SourceProductBaseCode=CT
  Gain2 : Gain  Gain=2*pi
  Product5 : Product
  Shapeit Integrator (Tustin) : Subsystem
  Shapeit Lead-Lag (Tustin) : Subsystem
  Out : Outport
  wires:
  In/1 -> Product5/1
  Shapeit Lead-Lag (Tustin)/1(Out) -> Discrete Varying Lowpass3/1
  Bus Selector/3 -> Shapeit Lead-Lag (Tustin)/2(fz)  "<LL_zero_fhz>"
  reset_integrator/1 -> Shapeit Integrator (Tustin)/3(reset)
  Bus Selector/4 -> Shapeit Lead-Lag (Tustin)/3(fp)  "<LL_pole_fhz>"
  Bus Selector/5 -> Gain2/1  "<LPF_fhz>"
  param/1 -> Bus Selector/1
  Bus Selector/2 -> Shapeit Integrator (Tustin)/2(I_fhz)  "<I_freq_hz>"
  Bus Selector/1 -> Product5/2  "<P_gain>"
  Shapeit Integrator (Tustin)/1(Out) -> Shapeit Lead-Lag (Tustin)/1(In)
  Discrete Varying Lowpass3/1 -> Out/1
  Product5/1 -> Shapeit Integrator (Tustin)/1(In)
  Gain2/1 -> Discrete Varying Lowpass3/2

== system ROPOD_Control_SIM/RopodTorqueDistribution/wheel vel cntr/Wheels Velocity controller/G_I_LL_LPF Controller8 ==
  param : Inport
  In : Inport  Port=2
  reset_integrator : Inport  Port=3
  Bus Selector : BusSelector  OutputSignals=P_gain,I_freq_hz,LL_zero_fhz,LL_pole_fhz,LPF_fhz
  Discrete Varying Lowpass3 : cstblocks/Linear Parameter Varying/Discrete Varying Lowpass  N=1  w0=0  Ts=Ts
      settings: SourceProductName=Control System Toolbox  SourceProductBaseCode=CT
  Gain2 : Gain  Gain=2*pi
  Product5 : Product
  Shapeit Integrator (Tustin) : Subsystem
  Shapeit Lead-Lag (Tustin) : Subsystem
  Out : Outport
  wires:
  Gain2/1 -> Discrete Varying Lowpass3/2
  Product5/1 -> Shapeit Integrator (Tustin)/1(In)
  Discrete Varying Lowpass3/1 -> Out/1
  Shapeit Integrator (Tustin)/1(Out) -> Shapeit Lead-Lag (Tustin)/1(In)
  Bus Selector/1 -> Product5/2  "<P_gain>"
  Bus Selector/2 -> Shapeit Integrator (Tustin)/2(I_fhz)  "<I_freq_hz>"
  param/1 -> Bus Selector/1
  Bus Selector/5 -> Gain2/1  "<LPF_fhz>"
  Bus Selector/4 -> Shapeit Lead-Lag (Tustin)/3(fp)  "<LL_pole_fhz>"
  reset_integrator/1 -> Shapeit Integrator (Tustin)/3(reset)
  Bus Selector/3 -> Shapeit Lead-Lag (Tustin)/2(fz)  "<LL_zero_fhz>"
  Shapeit Lead-Lag (Tustin)/1(Out) -> Discrete Varying Lowpass3/1
  In/1 -> Product5/1

== system ROPOD_Control_SIM/RopodVelocityController/Platorm Velocity controller/G_I_LL_LPF Controller_X/Shapeit Integrator (Tustin) ==
  In : Inport
  I_fhz : Inport  Port=2
  reset : Inport  Port=3
  Constant : Constant  Value=0
  Constant4 : Constant
  Constant5 : Constant  Value=0
  Gain2 : Gain  Gain=2*pi
  PID Controller3 : simulink/Continuous/PID Controller  Controller=PID  TimeDomain=Discrete-time  SampleTime=Ts  IntegratorMethod=Trapezoidal  FilterMethod=Trapezoidal  Form=Parallel  UseFilter=on  ControllerParametersSource=external  P=0.4  I=0.4*2*pi*3  D=0  N=100  InitialConditionSource=internal  InitialConditionForIntegrator=0  InitialConditionForFilter=0  ExternalReset=level  LimitOutput=on  UpperSaturationLimit=max_ropod_sw_force  LowerSaturationLimit=-max_ropod_sw_force  LinearizeAsGain=on  AntiWindupMode=clamping  Kb=1  TrackingMode=off  Kt=1  PParamMin=[]  PParamMax=[]  IParamMin=[]  IParamMax=[]  DParamMin=[]  DParamMax=[]  NParamMin=[]  NParamMax=[]  KbParamMin=[]  KbParamMax=[]  KtParamMin=[]  KtParamMax=[]  POutMin=[]  POutMax=[]  IOutMin=[]  IOutMax=[]  DOutMin=[]  DOutMax=[]  NOutMin=[]  NOutMax=[]  KbOutMin=[]  KbOutMax=[]  KtOutMin=[]  KtOutMax=[]  IntegratorOutMin=[]  IntegratorOutMax=[]  FilterOutMin=[]  FilterOutMax=[]  SumOutMin=[]  SumOutMax=[]  SumI1OutMin=[]  SumI1OutMax=[]  SumI2OutMin=[]  SumI2OutMax=[]  SumI3OutMin=[]  SumI3OutMax=[]  SumDOutMin=[]  SumDOutMax=[]  SaturationOutMin=[]  SaturationOutMax=[]  IntegratorContinuousStateAttributes=''  IntegratorStateMustResolveToSignalObject=off  IntegratorRTWStateStorageClass=Auto  FilterContinuousStateAttributes=''  FilterStateMustResolveToSignalObject=off  FilterRTWStateStorageClass=Auto  DifferentiatorICPrevScaledInput=0  DifferentiatorOutMin=[]  DifferentiatorOutMax=[]  InitialConditionSetting=State (most efficient)  FilterDiffOutCoefMin=[]  FilterDiffOutCoefMax=[]  SumDenOutMin=[]  SumDenOutMax=[]  SumNumOutMin=[]  SumNumOutMax=[]  ReciprocalOutMin=[]  ReciprocalOutMax=[]  DivideOutMin=[]  DivideOutMax=[]  TunerSelectOption=Transfer Function Based (PID Tuner App)
  Product4 : Product
  Out : Outport
  wires:
  I_fhz/1 -> Product4/2
  Product4/1 -> Gain2/1
  reset/1 -> PID Controller3/6
  Gain2/1 -> PID Controller3/3
  In/1 -> PID Controller3/1
  Constant4/1 -> Product4/1, PID Controller3/2
  Constant5/1 -> PID Controller3/5
  Constant/1 -> PID Controller3/4
  PID Controller3/1 -> Out/1

== system ROPOD_Control_SIM/RopodVelocityController/Platorm Velocity controller/G_I_LL_LPF Controller_X/Shapeit Lead-Lag (Tustin) ==
  In : Inport
  fz : Inport  Port=2
  fp : Inport  Port=3
  Add : Sum  Inputs=+-
  Constant1 : Constant
  Constant2 : Constant  Value=0
  Constant4 : Constant
  Divide : Product  Inputs=*/
  Divide1 : Product  Inputs=/*
  Gain1 : Gain  Gain=2*pi
  Gain2 : Gain  Gain=2*pi
  PID Controller3 : simulink/Continuous/PID Controller  Controller=PID  TimeDomain=Discrete-time  SampleTime=Ts  IntegratorMethod=Trapezoidal  FilterMethod=Trapezoidal  Form=Parallel  UseFilter=on  ControllerParametersSource=external  P=0.4  I=0.4*2*pi*3  D=0  N=100  InitialConditionSource=internal  InitialConditionForIntegrator=0  InitialConditionForFilter=0  ExternalReset=none  LimitOutput=off  UpperSaturationLimit=max_hw_tau  LowerSaturationLimit=-max_hw_tau  LinearizeAsGain=on  AntiWindupMode=clamping  Kb=1  TrackingMode=off  Kt=1  PParamMin=[]  PParamMax=[]  IParamMin=[]  IParamMax=[]  DParamMin=[]  DParamMax=[]  NParamMin=[]  NParamMax=[]  KbParamMin=[]  KbParamMax=[]  KtParamMin=[]  KtParamMax=[]  POutMin=[]  POutMax=[]  IOutMin=[]  IOutMax=[]  DOutMin=[]  DOutMax=[]  NOutMin=[]  NOutMax=[]  KbOutMin=[]  KbOutMax=[]  KtOutMin=[]  KtOutMax=[]  IntegratorOutMin=[]  IntegratorOutMax=[]  FilterOutMin=[]  FilterOutMax=[]  SumOutMin=[]  SumOutMax=[]  SumI1OutMin=[]  SumI1OutMax=[]  SumI2OutMin=[]  SumI2OutMax=[]  SumI3OutMin=[]  SumI3OutMax=[]  SumDOutMin=[]  SumDOutMax=[]  SaturationOutMin=[]  SaturationOutMax=[]  IntegratorContinuousStateAttributes=''  IntegratorStateMustResolveToSignalObject=off  IntegratorRTWStateStorageClass=Auto  FilterContinuousStateAttributes=''  FilterStateMustResolveToSignalObject=off  FilterRTWStateStorageClass=Auto  DifferentiatorICPrevScaledInput=0  DifferentiatorOutMin=[]  DifferentiatorOutMax=[]  InitialConditionSetting=State (most efficient)  FilterDiffOutCoefMin=[]  FilterDiffOutCoefMax=[]  SumDenOutMin=[]  SumDenOutMax=[]  SumNumOutMin=[]  SumNumOutMax=[]  ReciprocalOutMin=[]  ReciprocalOutMax=[]  DivideOutMin=[]  DivideOutMax=[]  TunerSelectOption=Transfer Function Based (PID Tuner App)
  Out : Outport
  wires:
  Constant4/1 -> PID Controller3/2
  In/1 -> PID Controller3/1
  PID Controller3/1 -> Out/1
  fz/1 -> Gain2/1
  fp/1 -> Gain1/1
  Gain1/1 -> PID Controller3/5, Divide/2
  Constant2/1 -> PID Controller3/3
  Gain2/1 -> Divide1/1, Divide/1
  Divide/1 -> Add/2
  Constant1/1 -> Add/1
  Add/1 -> Divide1/2
  Divide1/1 -> PID Controller3/4

== system ROPOD_Control_SIM/RopodVelocityController/Platorm Velocity controller/G_I_LL_LPF Controller_Y/Shapeit Integrator (Tustin) ==
  In : Inport
  I_fhz : Inport  Port=2
  reset : Inport  Port=3
  Constant : Constant  Value=0
  Constant4 : Constant
  Constant5 : Constant  Value=0
  Gain2 : Gain  Gain=2*pi
  PID Controller3 : simulink/Continuous/PID Controller  Controller=PID  TimeDomain=Discrete-time  SampleTime=Ts  IntegratorMethod=Trapezoidal  FilterMethod=Trapezoidal  Form=Parallel  UseFilter=on  ControllerParametersSource=external  P=0.4  I=0.4*2*pi*3  D=0  N=100  InitialConditionSource=internal  InitialConditionForIntegrator=0  InitialConditionForFilter=0  ExternalReset=level  LimitOutput=on  UpperSaturationLimit=max_ropod_sw_force  LowerSaturationLimit=-max_ropod_sw_force  LinearizeAsGain=on  AntiWindupMode=clamping  Kb=1  TrackingMode=off  Kt=1  PParamMin=[]  PParamMax=[]  IParamMin=[]  IParamMax=[]  DParamMin=[]  DParamMax=[]  NParamMin=[]  NParamMax=[]  KbParamMin=[]  KbParamMax=[]  KtParamMin=[]  KtParamMax=[]  POutMin=[]  POutMax=[]  IOutMin=[]  IOutMax=[]  DOutMin=[]  DOutMax=[]  NOutMin=[]  NOutMax=[]  KbOutMin=[]  KbOutMax=[]  KtOutMin=[]  KtOutMax=[]  IntegratorOutMin=[]  IntegratorOutMax=[]  FilterOutMin=[]  FilterOutMax=[]  SumOutMin=[]  SumOutMax=[]  SumI1OutMin=[]  SumI1OutMax=[]  SumI2OutMin=[]  SumI2OutMax=[]  SumI3OutMin=[]  SumI3OutMax=[]  SumDOutMin=[]  SumDOutMax=[]  SaturationOutMin=[]  SaturationOutMax=[]  IntegratorContinuousStateAttributes=''  IntegratorStateMustResolveToSignalObject=off  IntegratorRTWStateStorageClass=Auto  FilterContinuousStateAttributes=''  FilterStateMustResolveToSignalObject=off  FilterRTWStateStorageClass=Auto  DifferentiatorICPrevScaledInput=0  DifferentiatorOutMin=[]  DifferentiatorOutMax=[]  InitialConditionSetting=State (most efficient)  FilterDiffOutCoefMin=[]  FilterDiffOutCoefMax=[]  SumDenOutMin=[]  SumDenOutMax=[]  SumNumOutMin=[]  SumNumOutMax=[]  ReciprocalOutMin=[]  ReciprocalOutMax=[]  DivideOutMin=[]  DivideOutMax=[]  TunerSelectOption=Transfer Function Based (PID Tuner App)
  Product4 : Product
  Out : Outport
  wires:
  I_fhz/1 -> Product4/2
  Product4/1 -> Gain2/1
  reset/1 -> PID Controller3/6
  Gain2/1 -> PID Controller3/3
  PID Controller3/1 -> Out/1
  In/1 -> PID Controller3/1
  Constant4/1 -> Product4/1, PID Controller3/2
  Constant5/1 -> PID Controller3/5
  Constant/1 -> PID Controller3/4

== system ROPOD_Control_SIM/RopodVelocityController/Platorm Velocity controller/G_I_LL_LPF Controller_Y/Shapeit Lead-Lag (Tustin) ==
  In : Inport
  fz : Inport  Port=2
  fp : Inport  Port=3
  Add : Sum  Inputs=+-
  Constant1 : Constant
  Constant2 : Constant  Value=0
  Constant4 : Constant
  Divide : Product  Inputs=*/
  Divide1 : Product  Inputs=/*
  Gain1 : Gain  Gain=2*pi
  Gain2 : Gain  Gain=2*pi
  PID Controller3 : simulink/Continuous/PID Controller  Controller=PID  TimeDomain=Discrete-time  SampleTime=Ts  IntegratorMethod=Trapezoidal  FilterMethod=Trapezoidal  Form=Parallel  UseFilter=on  ControllerParametersSource=external  P=0.4  I=0.4*2*pi*3  D=0  N=100  InitialConditionSource=internal  InitialConditionForIntegrator=0  InitialConditionForFilter=0  ExternalReset=none  LimitOutput=off  UpperSaturationLimit=max_hw_tau  LowerSaturationLimit=-max_hw_tau  LinearizeAsGain=on  AntiWindupMode=clamping  Kb=1  TrackingMode=off  Kt=1  PParamMin=[]  PParamMax=[]  IParamMin=[]  IParamMax=[]  DParamMin=[]  DParamMax=[]  NParamMin=[]  NParamMax=[]  KbParamMin=[]  KbParamMax=[]  KtParamMin=[]  KtParamMax=[]  POutMin=[]  POutMax=[]  IOutMin=[]  IOutMax=[]  DOutMin=[]  DOutMax=[]  NOutMin=[]  NOutMax=[]  KbOutMin=[]  KbOutMax=[]  KtOutMin=[]  KtOutMax=[]  IntegratorOutMin=[]  IntegratorOutMax=[]  FilterOutMin=[]  FilterOutMax=[]  SumOutMin=[]  SumOutMax=[]  SumI1OutMin=[]  SumI1OutMax=[]  SumI2OutMin=[]  SumI2OutMax=[]  SumI3OutMin=[]  SumI3OutMax=[]  SumDOutMin=[]  SumDOutMax=[]  SaturationOutMin=[]  SaturationOutMax=[]  IntegratorContinuousStateAttributes=''  IntegratorStateMustResolveToSignalObject=off  IntegratorRTWStateStorageClass=Auto  FilterContinuousStateAttributes=''  FilterStateMustResolveToSignalObject=off  FilterRTWStateStorageClass=Auto  DifferentiatorICPrevScaledInput=0  DifferentiatorOutMin=[]  DifferentiatorOutMax=[]  InitialConditionSetting=State (most efficient)  FilterDiffOutCoefMin=[]  FilterDiffOutCoefMax=[]  SumDenOutMin=[]  SumDenOutMax=[]  SumNumOutMin=[]  SumNumOutMax=[]  ReciprocalOutMin=[]  ReciprocalOutMax=[]  DivideOutMin=[]  DivideOutMax=[]  TunerSelectOption=Transfer Function Based (PID Tuner App)
  Out : Outport
  wires:
  Constant4/1 -> PID Controller3/2
  In/1 -> PID Controller3/1
  PID Controller3/1 -> Out/1
  fz/1 -> Gain2/1
  fp/1 -> Gain1/1
  Gain1/1 -> PID Controller3/5, Divide/2
  Constant2/1 -> PID Controller3/3
  Gain2/1 -> Divide1/1, Divide/1
  Divide/1 -> Add/2
  Constant1/1 -> Add/1
  Add/1 -> Divide1/2
  Divide1/1 -> PID Controller3/4

== system ROPOD_Control_SIM/RopodVelocityController/Platorm Velocity controller/G_I_LL_LPF Controller_theta/Shapeit Integrator (Tustin) ==
  In : Inport
  I_fhz : Inport  Port=2
  reset : Inport  Port=3
  Constant : Constant  Value=0
  Constant4 : Constant
  Constant5 : Constant  Value=0
  Gain2 : Gain  Gain=2*pi
  PID Controller3 : simulink/Continuous/PID Controller  Controller=PID  TimeDomain=Discrete-time  SampleTime=Ts  IntegratorMethod=Trapezoidal  FilterMethod=Trapezoidal  Form=Parallel  UseFilter=on  ControllerParametersSource=external  P=0.4  I=0.4*2*pi*3  D=0  N=100  InitialConditionSource=internal  InitialConditionForIntegrator=0  InitialConditionForFilter=0  ExternalReset=level  LimitOutput=on  UpperSaturationLimit=max_ropod_sw_tau  LowerSaturationLimit=-max_ropod_sw_tau  LinearizeAsGain=on  AntiWindupMode=clamping  Kb=1  TrackingMode=off  Kt=1  PParamMin=[]  PParamMax=[]  IParamMin=[]  IParamMax=[]  DParamMin=[]  DParamMax=[]  NParamMin=[]  NParamMax=[]  KbParamMin=[]  KbParamMax=[]  KtParamMin=[]  KtParamMax=[]  POutMin=[]  POutMax=[]  IOutMin=[]  IOutMax=[]  DOutMin=[]  DOutMax=[]  NOutMin=[]  NOutMax=[]  KbOutMin=[]  KbOutMax=[]  KtOutMin=[]  KtOutMax=[]  IntegratorOutMin=[]  IntegratorOutMax=[]  FilterOutMin=[]  FilterOutMax=[]  SumOutMin=[]  SumOutMax=[]  SumI1OutMin=[]  SumI1OutMax=[]  SumI2OutMin=[]  SumI2OutMax=[]  SumI3OutMin=[]  SumI3OutMax=[]  SumDOutMin=[]  SumDOutMax=[]  SaturationOutMin=[]  SaturationOutMax=[]  IntegratorContinuousStateAttributes=''  IntegratorStateMustResolveToSignalObject=off  IntegratorRTWStateStorageClass=Auto  FilterContinuousStateAttributes=''  FilterStateMustResolveToSignalObject=off  FilterRTWStateStorageClass=Auto  DifferentiatorICPrevScaledInput=0  DifferentiatorOutMin=[]  DifferentiatorOutMax=[]  InitialConditionSetting=State (most efficient)  FilterDiffOutCoefMin=[]  FilterDiffOutCoefMax=[]  SumDenOutMin=[]  SumDenOutMax=[]  SumNumOutMin=[]  SumNumOutMax=[]  ReciprocalOutMin=[]  ReciprocalOutMax=[]  DivideOutMin=[]  DivideOutMax=[]  TunerSelectOption=Transfer Function Based (PID Tuner App)
  Product4 : Product
  Out : Outport
  wires:
  I_fhz/1 -> Product4/2
  Product4/1 -> Gain2/1
  reset/1 -> PID Controller3/6
  Gain2/1 -> PID Controller3/3
  PID Controller3/1 -> Out/1
  In/1 -> PID Controller3/1
  Constant4/1 -> Product4/1, PID Controller3/2
  Constant5/1 -> PID Controller3/5
  Constant/1 -> PID Controller3/4
